simulink model "UNICON_longi_total"  (R2025b)
settings: Solver=ode4  StartTime=0  StopTime=840  FixedStep=0.001  RelTol=1e-3  EnableMultiTasking=on
libraries: Solver_SF x2
settings Model: ExtModeTrigMode=oneshot  ExtModeArmWhenConnect=off  Creator=dhall  LastModifiedBy=user
settings SolverCC: AlgebraicLoopSolver=TrustRegion  AutoInsertRateTranBlk=on
settings DataIOCC: SaveFormat=Array  SignalLoggingSaveFormat=ModelDataLogs  ReturnWorkspaceOutputs=off  SignalLoggingName=sigsOut
settings OptimizationCC: BooleanDataType=off  LocalBlockOutputs=off  InitFltsAndDblsToZero=on  LifeSpan=inf
settings DebuggingCC: SaveWithParameterizedLinksMsg=none  UnderspecifiedInitializationDetection=Classic  MergeDetectMultiDrivingBlocksExec=none  SignalResolutionControl=TryResolveAllWithWarning  MultiTaskDSMMsg=warning  MultiTaskCondExecSysMsg=none  FcnCallInpInsideContextMsg=warning  UnconnectedInputMsg=warning  UnconnectedOutputMsg=warning  UnconnectedLineMsg=warning  StateNameClashWarn=warning  SFUnexpectedBacktrackingDiag=warning  SFNoUnconditionalDefaultTransitionDiag=warning  SFExecutionAtInitializationDiag=none  ArithmeticOperatorsInVariantConditions=warning
settings HardwareCC: TargetBitPerPointer=64.0  TargetBitPerSizeT=64.0  TargetBitPerPtrDiffT=64.0  TargetLongLongMode=on  TargetIntDivRoundTo=Zero  TargetEndianess=LittleEndian  TargetWordSize=64.0  TargetPreprocMaxBitsSint=64.0  TargetPreprocMaxBitsUint=64.0  TargetHWDeviceType=MATLAB Host  ProdEqTarget=off
settings ModelReferenceCC: EnableRefExpFcnMdlSchedulingChecks=on  PropagateSignalLabelsOutOfModel=off
settings SFSimCC: SimUseLocalCustomCode=off  CustomCodeUndefinedFunction=UseInterfaceOnly
settings RTWCC: RTWUseLocalCustomCode=off  GPUComputeCapability=3.5  DLArmComputeVersion=19.05
settings CodeAppCC: StateflowObjectComments=on
settings GRTTargetCC: TargetFcnLib=ansi_tfl_tmw.mat  TargetLangStandard=C89/C90 (ANSI)  CompOptLevelCompliant=off  CombineOutputUpdateFcns=off  GRTInterface=on
settings ConfigComp: CovMetricSettings=dw  CovSaveCumulativeToWorkspaceVar=on  CovSaveSingleToWorkspaceVar=on  CovExternalEMLEnable=off

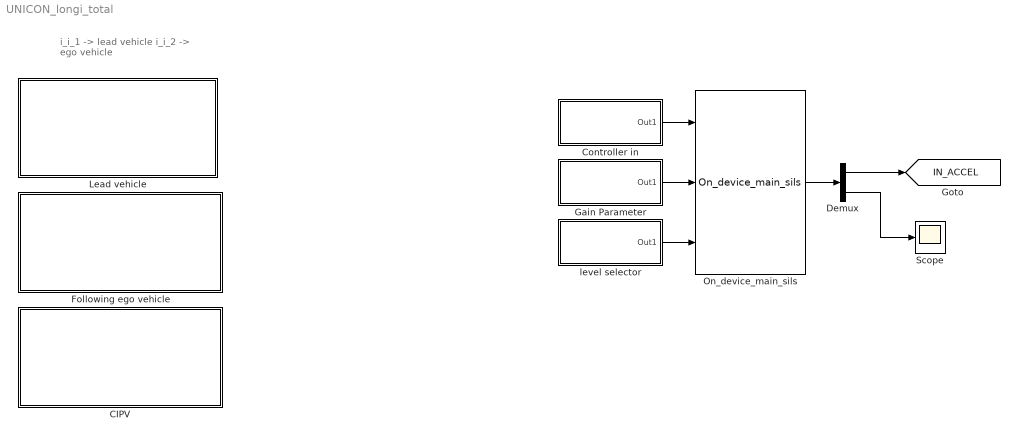
== system UNICON_longi_total ==
  note: i_i_1 -> lead vehicle
      | i_i_2 -> ego vehicle
  CIPV : Subsystem
  Controller in : Subsystem
  Demux : Demux  Outputs=2
  Following ego vehicle : Subsystem
  Gain Parameter : Subsystem
  Lead vehicle : Subsystem
  On_device_main_sils : S-Function  FunctionName=On_device_main_sils  SFunctionDeploymentMode=off  EnableBusSupport=off
      mask Display: disp('Controller')
  Scope : Scope
      settings: ActiveDisplayYMinimum=-0.12499999999999997  ActiveDisplayYMaximum=1.125  DataLoggingVariableName=ScopeData8
  level selector : Subsystem
  tag scope: IN_ACCEL=global
  wires:
  Gain Parameter/1(Out1) -> On_device_main_sils/2
  level selector/1(Out1) -> On_device_main_sils/3
  Controller in/1(Out1) -> On_device_main_sils/1
  On_device_main_sils/1 -> Demux/1
  Demux/1 -> [IN_ACCEL]
  Demux/2 -> Scope/1

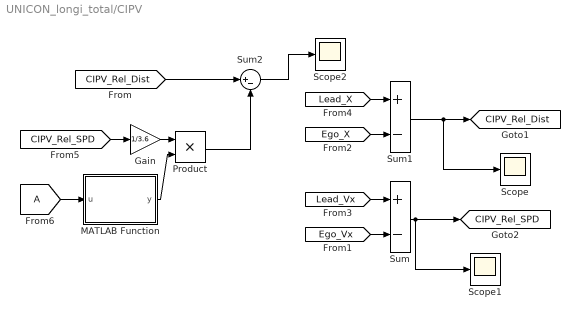
== system UNICON_longi_total/CIPV ==
  From6 : From  TagVisibility=global
  Gain : Gain  Gain=1/3.6
  MATLAB Function : MATLAB Function  TreatAsAtomicUnit=on
  Product : Product
  Scope : Scope
      settings: ActiveDisplayYMinimum=14.164049582686104  ActiveDisplayYMaximum=112.24186908286582  DataLoggingVariableName=ScopeData9
  Scope1 : Scope
      settings: ActiveDisplayYMinimum=-12.498874521115376  ActiveDisplayYMaximum=12.499874946790596  DataLoggingVariableName=ScopeData10
  Scope2 : Scope
      settings: ActiveDisplayYMinimum=-13.119566925749361  ActiveDisplayYMaximum=118.07610233174428  DataLoggingVariableName=ScopeData16
  Sum : Sum  Inputs=+-
  Sum1 : Sum  Inputs=+-
  Sum2 : Sum  Inputs=|+-
  tag scope: CIPV_Rel_Dist=global, CIPV_Rel_SPD=global
  wires:
  [Ego_Vx] -> Sum/2
  [Lead_Vx] -> Sum/1
  [Ego_X] -> Sum1/2
  [Lead_X] -> Sum1/1
  Sum1/1 -> Scope/1, [CIPV_Rel_Dist]
  Sum/1 -> Scope1/1, [CIPV_Rel_SPD]
  From6/1 -> MATLAB Function/1(u)
  MATLAB Function/1(y) -> Product/2
  [CIPV_Rel_Dist] -> Sum2/1
  Product/1 -> Sum2/2
  Sum2/1 -> Scope2/1
  [CIPV_Rel_SPD] -> Gain/1
  Gain/1 -> Product/1

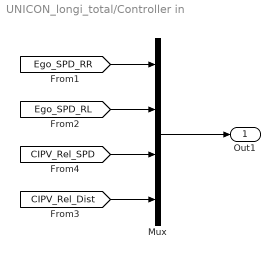
== system UNICON_longi_total/Controller in ==
  Mux : Mux
  Out1 : Outport
  wires:
  Mux/1 -> Out1/1
  [Ego_SPD_RR] -> Mux/1
  [Ego_SPD_RL] -> Mux/2
  [CIPV_Rel_SPD] -> Mux/3
  [CIPV_Rel_Dist] -> Mux/4

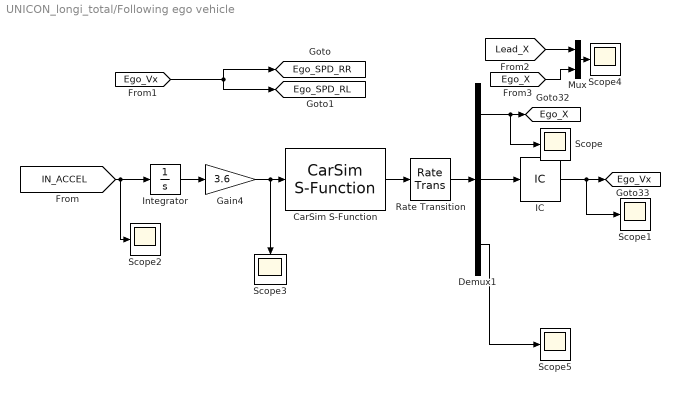
== system UNICON_longi_total/Following ego vehicle ==
  CarSim S-Function : Solver_SF/CarSim S-Function  Priority=1  VehicleCode=i_i_2  SIMFILE=simfile2.sim
  Demux1 : Demux  Outputs=3
  Gain4 : Gain  Gain=3.6
  IC : InitialCondition  Value=40
  Integrator : Integrator  InitialCondition=40/3.6
  Mux : Mux  Inputs=2
  Rate Transition : RateTransition  Integrity=off  OutPortSampleTime=Tc
  Scope{,1..5} (6 alike) : Scope
      Scope settings: ActiveDisplayYMinimum=-341.98541722478797  ActiveDisplayYMaximum=3077.868755023092  DataLoggingVariableName=ScopeData3
      Scope1 settings: ActiveDisplayYMinimum=30.759412325086878  ActiveDisplayYMaximum=69.166049222661925  DataLoggingVariableName=ScopeData4
      Scope2 settings: ActiveDisplayYMinimum=-3.75  ActiveDisplayYMaximum=3.75  DataLoggingVariableName=ScopeData5
      Scope3 settings: ActiveDisplayYMinimum=14.296294583773298  ActiveDisplayYMaximum=87.99252050929671
      Scope4 settings: ActiveDisplayYMinimum=-877.01581281967128  ActiveDisplayYMaximum=7893.1423153770438  DataLoggingVariableName=ScopeData7
      Scope5 settings: ActiveDisplayYMinimum=-1  ActiveDisplayYMaximum=1  DataLoggingVariableName=ScopeData13
  tag scope: Ego_SPD_RL=global, Ego_SPD_RR=global, Ego_Vx=global, Ego_X=global
  wires:
  Gain4/1 -> CarSim S-Function/1, Scope3/1
  Integrator/1 -> Gain4/1
  [IN_ACCEL] -> Integrator/1, Scope2/1
  CarSim S-Function/1 -> Rate Transition/1
  Demux1/1 -> Scope/1, [Ego_X]
  Rate Transition/1 -> Demux1/1
  [Ego_Vx] -> [Ego_SPD_RR], [Ego_SPD_RL]
  [Lead_X] -> Mux/1
  [Ego_X] -> Mux/2
  Mux/1 -> Scope4/1
  Demux1/3 -> Scope5/1
  IC/1 -> Scope1/1, [Ego_Vx]
  Demux1/2 -> IC/1

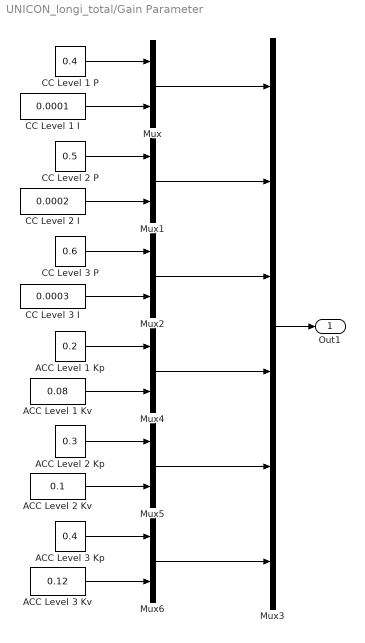
== system UNICON_longi_total/Gain Parameter ==
  ACC Level 1 Kp : Constant  Value=0.2
  ACC Level 1 Kv : Constant  Value=0.08
  ACC Level 2 Kp : Constant  Value=0.3
  ACC Level 2 Kv : Constant  Value=0.1
  ACC Level 3 Kp : Constant  Value=0.4
  ACC Level 3 Kv : Constant  Value=0.12
  CC Level 1 I : Constant  Value=0.0001
  CC Level 1 P : Constant  Value=0.4
  CC Level 2 I : Constant  Value=0.0002
  CC Level 2 P : Constant  Value=0.5
  CC Level 3 I : Constant  Value=0.0003
  CC Level 3 P : Constant  Value=0.6
  Mux{,1..2,4..6} (6 alike) : Mux  Inputs=2
  Mux3 : Mux  Inputs=6
  Out1 : Outport
  wires:
  Mux3/1 -> Out1/1
  CC Level 1 P/1 -> Mux/1
  CC Level 1 I/1 -> Mux/2
  CC Level 2 I/1 -> Mux1/2
  CC Level 2 P/1 -> Mux1/1
  CC Level 3 I/1 -> Mux2/2
  CC Level 3 P/1 -> Mux2/1
  ACC Level 1 Kv/1 -> Mux4/2
  ACC Level 1 Kp/1 -> Mux4/1
  ACC Level 2 Kv/1 -> Mux5/2
  ACC Level 2 Kp/1 -> Mux5/1
  ACC Level 3 Kv/1 -> Mux6/2
  ACC Level 3 Kp/1 -> Mux6/1
  Mux/1 -> Mux3/1
  Mux1/1 -> Mux3/2
  Mux2/1 -> Mux3/3
  Mux4/1 -> Mux3/4
  Mux5/1 -> Mux3/5
  Mux6/1 -> Mux3/6

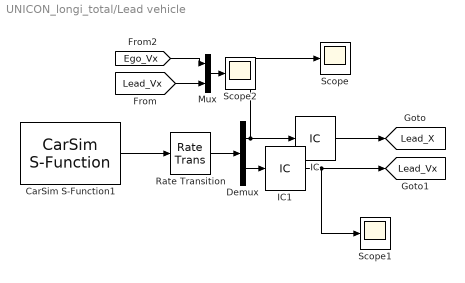
== system UNICON_longi_total/Lead vehicle ==
  CarSim S-Function1 : Solver_SF/CarSim S-Function  Priority=1  VehicleCode=i_i_1  SIMFILE=simfile1.sim
  Demux : Demux  Outputs=2
  IC : InitialCondition  Value=100
  IC1 : InitialCondition  Value=50
  Mux : Mux  Inputs=2
  Rate Transition : RateTransition  Integrity=off  OutPortSampleTime=Tc
  Scope : Scope
      settings: ActiveDisplayYMinimum=-533.29874386342988  ActiveDisplayYMaximum=4799.68869477087
  Scope1 : Scope
      settings: ActiveDisplayYMinimum=-5.3734251811760165  ActiveDisplayYMaximum=111.87745771809416  DataLoggingVariableName=ScopeData2
  Scope2 : Scope
      settings: ActiveDisplayYMinimum=-1  ActiveDisplayYMaximum=1  DataLoggingVariableName=ScopeData6
  tag scope: Lead_Vx=global, Lead_X=global
  wires:
  Rate Transition/1 -> Demux/1
  CarSim S-Function1/1 -> Rate Transition/1
  Demux/2 -> IC1/1
  Demux/1 -> Scope/1, IC/1
  IC/1 -> [Lead_X]
  IC1/1 -> Scope1/1, [Lead_Vx]
  [Lead_Vx] -> Mux/2
  [Ego_Vx] -> Mux/1
  Mux/1 -> Scope2/1

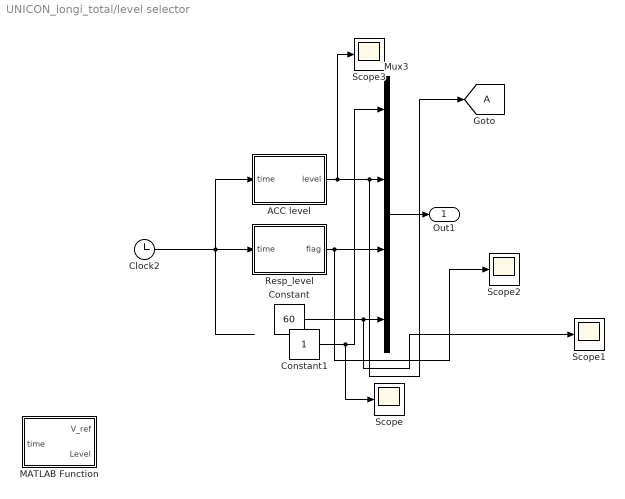
== system UNICON_longi_total/level selector ==
  ACC level : MATLAB Function  TreatAsAtomicUnit=on
  Clock2 : Clock
  Constant : Constant  Value=60
  Constant1 : Constant
  Goto : Goto  TagVisibility=global
  MATLAB Function : MATLAB Function  TreatAsAtomicUnit=on
  Mux3 : Mux
  Resp_level : MATLAB Function  TreatAsAtomicUnit=on
  Scope{,1..3} (4 alike) : Scope
      Scope settings: ActiveDisplayYMinimum=-1  ActiveDisplayYMaximum=1  DataLoggingVariableName=ScopeData11
      Scope1 settings: ActiveDisplayYMinimum=60  ActiveDisplayYMaximum=80  DataLoggingVariableName=ScopeData12
      Scope2 settings: ActiveDisplayYMinimum=0.75000000000000011  ActiveDisplayYMaximum=3.25  DataLoggingVariableName=ScopeData14
      Scope3 settings: ActiveDisplayYMinimum=0.75000000000000011  ActiveDisplayYMaximum=3.25  DataLoggingVariableName=ScopeData15
  Out1 : Outport
  wires:
  Mux3/1 -> Out1/1
  Resp_level/1(flag) -> Scope2/1, Mux3/3
  Clock2/1 -> ACC level/1(time), Resp_level/1(time)
  ACC level/1(level) -> Scope3/1, Goto/1, Mux3/2
  Constant/1 -> Scope1/1, Mux3/4
  Constant1/1 -> Scope/1, Mux3/1

== matlab function UNICON_longi_total/level selector/Resp_level ==
  data: time input; flag output
function flag = timeFlag(time)

    % 초기 30초 offset
    if time < 45
        flag = 1;

    % 이후 90초마다 Flag 변경
    else
        flag = mod(floor((time - 45) / 90), 3) + 1;
    end

end

== matlab function UNICON_longi_total/level selector/MATLAB Function ==
  data: time input; V_ref output; Level output
function [V_ref, Level] = CC_Profile(time)

    %% Level
    if time < 150
        Level = 1;
    elseif time < 300
        Level = 2;
    else
        Level = 3;
    end

    %% Local time for each Level
    t = mod(time,150);

    %% Target speed
    if t < 30
        V_ref = 50;

    elseif t < 60
        V_ref = 65;

    elseif t < 90
        V_ref = 50;

    elseif t < 120
        V_ref = 35;

    else
        V_ref = 50;
    end

end

== matlab function UNICON_longi_total/CIPV/MATLAB Function ==
  data: u input; y output
function y = fcn(u)

if u == 1
    y = 2.5;
elseif u == 2
    y = 3.5;
else
    y = 4.5;
end

== matlab function UNICON_longi_total/level selector/ACC level ==
  data: time input; level output
function level = levelselect(time)

    if time < 315
        level = 1;

    elseif time < 585
        level = 2;

    elseif time < 855
        level = 3;

    else
        level = 1;
    end

end
